simulink model "pseudo_derivative_model"  (R2016b)
settings: Solver=ode3  StartTime=0.0  StopTime=t_final  FixedStep=T  RelTol=1e-3  EnableMultiTasking=on
values from neighbouring files (symbols this model uses):
  a = 100    [MAIN_pseudo_derivative.m]
  noise_amplitude = 0.05    [MAIN_pseudo_derivative.m]
  T = 0.001    [MAIN_pseudo_derivative.m]
  w_e = 1    [MAIN_pseudo_derivative.m]
settings Model: Creator=lum  LastModifiedBy=Christopher
settings DataIOCC: LimitDataPoints=on  SaveFormat=Array  SignalLoggingSaveFormat=ModelDataLogs
settings OptimizationCC: ExpressionDepthLimit=2147483647  LifeSpan=inf
settings DebuggingCC: UnderspecifiedInitializationDetection=Classic  MergeDetectMultiDrivingBlocksExec=none  SolverPrmCheckMsg=warning  FcnCallInpInsideContextMsg=warning  AllowSymbolicDim=off  StateNameClashWarn=warning  SFUnexpectedBacktrackingDiag=warning  SFNoUnconditionalDefaultTransitionDiag=warning  SFExecutionAtInitializationDiag=none
settings HardwareCC: ProdBitPerPointer=32  ProdBitPerSizeT=32  ProdBitPerPtrDiffT=32  ProdLargestAtomicFloat=None  ProdIntDivRoundTo=Undefined  ProdEndianess=Unspecified  ProdWordSize=32  ProdHWDeviceType=32-bit Generic
settings ModelReferenceCC: PropagateSignalLabelsOutOfModel=off
settings GRTTargetCC: TargetLangStandard=C89/C90 (ANSI)  GeneratePreprocessorConditionals=Disable all  CombineOutputUpdateFcns=off  GRTInterface=on
settings ConfigComp: CovMetricSettings=dw  CovHtmlReporting=on  CovSaveCumulativeToWorkspaceVar=on  CovSaveSingleToWorkspaceVar=on  CovExternalEMLEnable=off

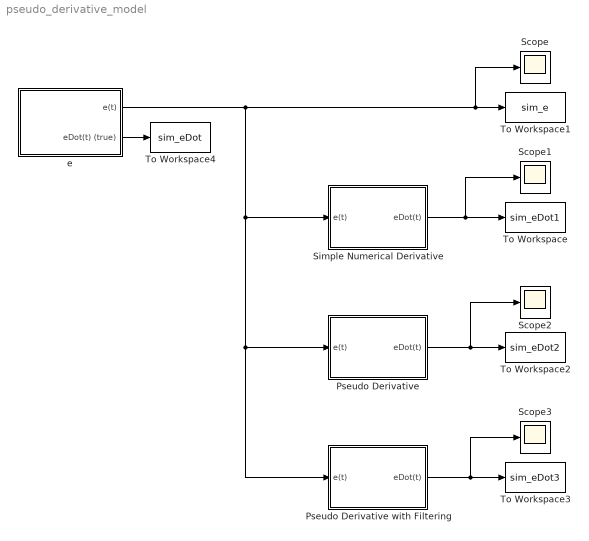
== system pseudo_derivative_model ==
  Pseudo Derivative : Subsystem
  Pseudo Derivative with Filtering : Subsystem
  Scope{,1..3} (4 alike) : Scope
  Simple Numerical Derivative : Subsystem
  To Workspace : ToWorkspace  VariableName=sim_eDot1  SaveFormat=Structure With Time  SampleTime=-1
  To Workspace1 : ToWorkspace  VariableName=sim_e  SaveFormat=Structure With Time  SampleTime=-1
  To Workspace2 : ToWorkspace  VariableName=sim_eDot2  SaveFormat=Structure With Time  SampleTime=-1
  To Workspace3 : ToWorkspace  VariableName=sim_eDot3  SaveFormat=Structure With Time  SampleTime=-1
  To Workspace4 : ToWorkspace  VariableName=sim_eDot  SaveFormat=Structure With Time  SampleTime=-1
  e : Subsystem
  wires:
  e/1(e(t)) -> Simple Numerical Derivative/1(e(t)), Pseudo Derivative/1(e(t)), Pseudo Derivative with Filtering/1(e(t)), To Workspace1/1, Scope/1
  Simple Numerical Derivative/1(eDot(t)) -> To Workspace/1, Scope1/1
  Pseudo Derivative/1(eDot(t)) -> To Workspace2/1, Scope2/1
  Pseudo Derivative with Filtering/1(eDot(t)) -> To Workspace3/1, Scope3/1
  e/2(eDot(t) (true)) -> To Workspace4/1

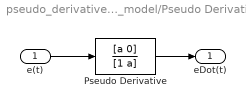
== system pseudo_derivative_model/Pseudo Derivative ==
  e(t) : Inport
  Pseudo Derivative : TransferFcn  Numerator=[a 0]  Denominator=[1 a]
  eDot(t) : Outport
  wires:
  Pseudo Derivative/1 -> eDot(t)/1
  e(t)/1 -> Pseudo Derivative/1

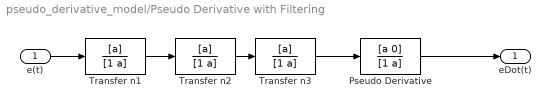
== system pseudo_derivative_model/Pseudo Derivative with Filtering ==
  e(t) : Inport
  Pseudo Derivative : TransferFcn  Numerator=[a 0]  Denominator=[1 a]
  Transfer n1 : TransferFcn  Numerator=[a]  Denominator=[1 a]
  Transfer n2 : TransferFcn  Numerator=[a]  Denominator=[1 a]
  Transfer n3 : TransferFcn  Numerator=[a]  Denominator=[1 a]
  eDot(t) : Outport
  wires:
  e(t)/1 -> Transfer n1/1
  Pseudo Derivative/1 -> eDot(t)/1
  Transfer n1/1 -> Transfer n2/1
  Transfer n2/1 -> Transfer n3/1
  Transfer n3/1 -> Pseudo Derivative/1

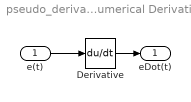
== system pseudo_derivative_model/Simple Numerical Derivative ==
  e(t) : Inport
  Derivative : Derivative
  eDot(t) : Outport
  wires:
  e(t)/1 -> Derivative/1
  Derivative/1 -> eDot(t)/1

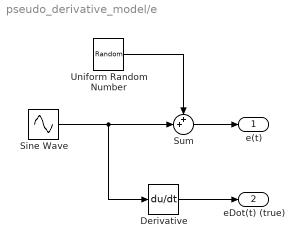
== system pseudo_derivative_model/e ==
  Derivative : Derivative
  Sine Wave : Sin  Frequency=w_e  SampleTime=0
  Sum : Sum  Inputs=++|
  Uniform Random Number : UniformRandomNumber  Minimum=-noise_amplitude  Maximum=noise_amplitude  SampleTime=T
  e(t) : Outport
  eDot(t) (true) : Outport  Port=2
  wires:
  Sum/1 -> e(t)/1
  Uniform Random Number/1 -> Sum/1
  Sine Wave/1 -> Sum/2, Derivative/1
  Derivative/1 -> eDot(t) (true)/1
